simulink model "Motor_DC_simu"  (R2022a)
settings: Solver=VariableStepAuto  StartTime=0.0  StopTime=10.0  RelTol=1e-3
values from neighbouring files (symbols this model uses):
  B = 12e-4    (= 0.0012)    [MotorDc_parametros_simu.m]
  J = 1e-3    (= 0.001)    [MotorDc_parametros_simu.m]
  Kt = 0.01    [MotorDc_parametros_simu.m]
  Kv = 0.01    [MotorDc_parametros_simu.m]
  L = 23e-3    (= 0.023)    [MotorDc_parametros_simu.m]
  R = 2    [MotorDc_parametros_simu.m]
undefined symbols (not defined in the file or in its folder): Vi
settings Model: Creator=ivsid  LastModifiedBy=ivsid

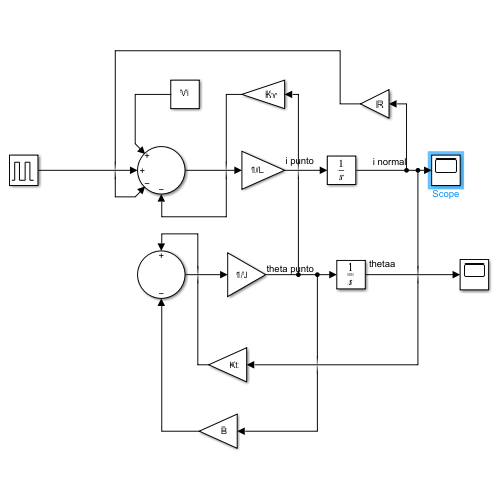
[thumbnail: Simulink's stored preview of the top-level diagram]
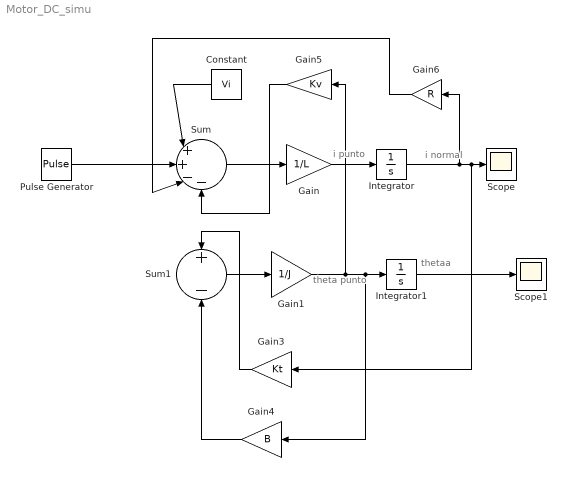
== system Motor_DC_simu ==
  note: thetaa
  note: theta punto
  note: i normal
  note: i punto
  Constant : Constant  Value=Vi
  Gain : Gain  Gain=1/L
  Gain1 : Gain  Gain=1/J
  Gain3 : Gain  Gain=Kt
  Gain4 : Gain  Gain=B
  Gain5 : Gain  Gain=Kv
  Gain6 : Gain  Gain=R
  Integrator : Integrator
  Integrator1 : Integrator
  Pulse Generator : DiscretePulseGenerator  PulseType=Time based  Amplitude=24  Period=1/20000  PulseWidth=25
  Scope : Scope
  Scope1 : Scope
  Sum : Sum  Inputs=|++--
  Sum1 : Sum  Inputs=+-
  wires:
  Sum/1 -> Gain/1
  Gain/1 -> Integrator/1
  Integrator/1 -> Gain6/1, Gain3/1, Scope/1
  Constant/1 -> Sum/1
  Integrator1/1 -> Scope1/1
  Gain3/1 -> Sum1/1
  Gain4/1 -> Sum1/2
  Sum1/1 -> Gain1/1
  Pulse Generator/1 -> Sum/2
  Gain1/1 -> Gain4/1, Integrator1/1, Gain5/1
  Gain5/1 -> Sum/4
  Gain6/1 -> Sum/3
